simulink model "ferranti3phaseupfc41"  (R2016a)
settings: Solver=VariableStepAuto  StartTime=0.0  StopTime=10.0  RelTol=1e-3
undefined symbols (not defined in the file): D1, Delta
libraries: powerlib x20, powerlib_meascontrol x5, sps_avr x2, factslib x1
settings Model: Creator=prajay  LastModifiedBy=prajay

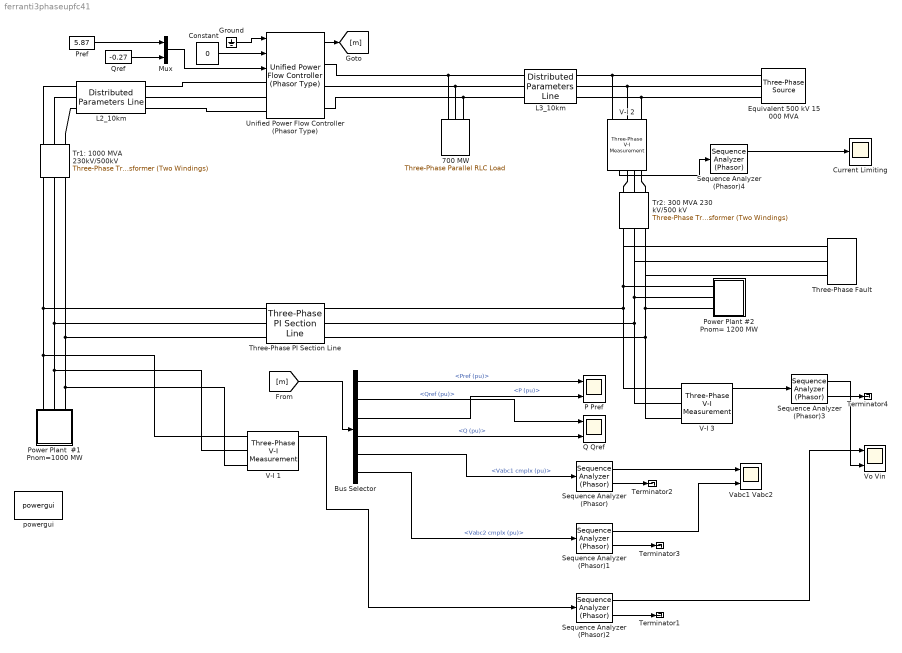
== system ferranti3phaseupfc41 ==
  700 MW : powerlib/Elements/Three-Phase Parallel RLC Load  LConnTagsString=A|B|C  Configuration=Y (grounded)  NominalVoltage=500e3  Vabc=[1e3 1e3 1e3]  Vabcp=[1e3 1e3 1e3]  NominalFrequency=60  UnbalancedPower=off  ActivePower=700e+006  InductivePower=0  CapacitivePower=0  Pabc=[10e3 9e3 11e3]  QLabc=[100 90 110]  QCabc=[100 90 110]  Pabcp=[10e3 9e3 11e3]  QLabcp=[100 90 110]  QCabcp=[100 90 110]  Measurements=None  LoadType=constant Z
  Bus Selector : BusSelector  OutputSignals=Control (Series).Pref (pu),Control (Series).Qref (pu),Control (Series).P (pu),Control (Series).Q (pu),Power.Vabc1 cmplx (pu),Power.Vabc2 cmplx (pu)
  Constant : Constant  Value=0
  Current Limiting : Scope
  Equivalent 500 kV 15 000 MVA : powerlib/Electrical Sources/Three-Phase Source  InternalConnection=Yg  VoltagePhases=off  Voltage=(500000)*1  PhaseAngle=3.2028e-005  Voltage_phases=[25e3 25e3 25e3]/sqrt(3)  PhaseAngles_phases=[0 -120 +120]  Frequency=60  NonIdealSource=on  SpecifyImpedance=on  Resistance=0.8929  Inductance=16.58e-3  ShortCircuitLevel=15000e6  BaseVoltage=500e3  XRratio=10  BusType=swing  Pref=0  Qref=0  Prefabc=0  Qrefabc=0  Qmin=-Inf  Qmax=Inf
  Ground : Ground
  L2_10km : powerlib/Elements/Distributed Parameters Line  Phases=3  Frequency=60  Resistance=[0.01273*2 0.3864]  Inductance="[0.9337e-3  4.1264e-3]"  Capacitance=[12.74e-9 7.751e-9]  Length=10  x1=[3.76470393664515e-08 500737.865699465 500737.698733622;376.991118430775 376.991118430775 376.991118430775;-1.76616198142372 0.572801869127968 -0.997994660183336]  x2=[3.31706486217144e-08 500303.506190995 500303.363079344;376.991118430775 376.991118430775 376.991118430775;-2.24825401600232 0.564569126636545 -1.00622737253496]  x3=[1.03911611711346e-09 676.330782319688 676.334945484693;376.991118430775 376.991118430775 376.991118430775;1.10566566451741 0.619123018648377 -0.951683326428739]  x4=[1.12477345287176e-09 3020.16196617448 3020.15620594757;376.991118430775 376.991118430775 376.991118430775;-2.03075400822802 0.549440453871556 -1.0213539651237]  x5=5.65541566995743e-05  V1=[3.169e-08 5.017e+05 5.017e+05;377 377 377;-0.2885 0.6054 -0.9654]  V2=[5.891e-08 5.011e+05 5.011e+05;377 377 377;2.202 0.568 -1.003]  I1=[1.07e-09 790.2 790.2;377 377 377;1.059 0.5023 -1.068]  I2=[1.028e-09 2904 2904;377 377 377;-2.11 0.5682 -1.003]  nHarmo=1  Measurements=Phase-to-ground voltages
      settings: AttributesFormatString=\n
  L3_10km : powerlib/Elements/Distributed Parameters Line  Phases=3  Frequency=60  Resistance=[0.01273*2 0.3864]  Inductance="[0.9337e-3  4.1264e-3]"  Capacitance=[12.74e-9 7.751e-9]  Length=10  x1=[3.32362335184301e-08 500303.388829253 500303.245718116;376.991118430775 376.991118430775 376.991118430775;-2.24805262409125 0.564569135773158 -1.00622736339962]  x2=[3.74559266249712e-08 500158.715856024 500158.596416031;376.991118430775 376.991118430775 376.991118430775;-2.6669204011152 0.566197665169602 -1.0045988035158]  x3=[9.25310885665503e-10 2074.37871582524 2074.38278202316;376.991118430775 376.991118430775 376.991118430775;1.21991146236643 0.586596456295587 -0.984203157060539]  x4=[9.8818528826696e-10 1620.48120507726 1620.47576843211;376.991118430775 376.991118430775 376.991118430775;-1.97224320713439 0.523398649863408 -1.04739401571321]  x5=5.65541566995743e-05  V1=[5.882e-08 5.011e+05 5.011e+05;377 377 377;2.203 0.568 -1.003]  V2=[1.45e-07 4.993e+05 4.993e+05;377 377 377;2.363 0.5448 -1.026]  I1=[1.123e-09 1185 1185;377 377 377;1.202 0.5674 -1.003]  I2=[1.02e-09 2501 2501;377 377 377;-2.175 0.5033 -1.068]  nHarmo=1  Measurements=None
      settings: AttributesFormatString=\n
  Mux : Mux  Inputs=2
  P Pref : Scope  NumInputPorts=2
  Power Plant  #1 Pnom=1000 MW : Subsystem
  Power Plant #2 Pnom= 1200 MW : Subsystem
  Pref : Constant  Value=5.87
  Q Qref : Scope  NumInputPorts=2
  Qref : Constant  Value=-0.27
  Sequence Analyzer (Phasor){,1..4} (5 alike) : powerlib_meascontrol/Measurements/Sequence Analyzer (Phasor)  seq=Positive
  Terminator{1..4} (4 alike) : Terminator
  Three-Phase PI Section Line : powerlib/Elements/Three-Phase PI Section Line  LConnTagsString=a|b|c  RConnTagsString=A|B|C  Frequency=60  Resistances=[ 0.01273 0.3864]  Inductances="[ 0.9337e-3  4.1264e-3]"  Capacitances=[12.74e-9 7.751e-9]  Length=800
  Three-Phase Fault : powerlib/Elements/Three-Phase Fault  InitialStates=0  FaultA=on  FaultB=on  FaultC=on  GroundFault=on  SwitchTimes="[1/60  5/60]"  External=off  SwitchStatus=NaN  FaultResistance=0.001  GroundResistance=0.01  SnubberResistance=1e6  SnubberCapacitance=inf  Measurements=None
  Tr1: 1000 MVA 230kV/500kV : powerlib/Elements/Three-Phase Transformer (Two Windings)  Winding1Connection=Yg  Winding2Connection=Yg  CoreType=Three single-phase transformers  SetSaturation=off  Hysteresis=off  DataFile='basic_model'  SetInitialFlux=off  Measurements=None  UNITS=pu  NominalPower=[ 1000e6 60 ]  Winding1="[ 230e3 0.002  0.0]"  Winding2=[ 500e3 0.002 0.12]  Rm=500  Lm=500  L0=0.5  Saturation="[ 0,0  ;  0.005,1.2  ;  1.0,1.4 ]"  InitialFluxes=[ 0.8 , -0.8 , 0.7 ]  MoreParameters=off  BreakLoop=off  DataType=off  TransfoNumber=0
  Tr2: 300 MVA 230 kV/500 kV : powerlib/Elements/Three-Phase Transformer (Two Windings)  Winding1Connection=Yg  Winding2Connection=Yg  CoreType=Three single-phase transformers  SetSaturation=off  Hysteresis=off  DataFile='basic_model'  SetInitialFlux=off  Measurements=Winding voltages  UNITS=pu  NominalPower=[ 300e6 60 ]  Winding1="[ 230e3 0.002  0.0]"  Winding2=[ 500e3 0.002 0.15]  Rm=500  Lm=500  L0=0.5  Saturation="[ 0,0  ;  0.005,1.2  ;  1.0,1.4 ]"  InitialFluxes=[ 0.8 , -0.8 , 0.7 ]  MoreParameters=off  BreakLoop=off  DataType=off  TransfoNumber=0
  Unified Power Flow Controller (Phasor Type) : factslib/Power-Electronics Based FACTS/Unified Power Flow Controller (Phasor Type)  SystemNominal=[ 500e3, 60 ]  Pnom_SH=100e6  RL_SH=[ 0.22/30, 0.22 ]  Iinit_SH=[0, 0 ]  SeriesNominal=[ 100e6, 0.1]  RL_SE=[ 0.16/30, 0.16 ]  Iinit_SE=[ 0 0]  VnomDC=40000  C_DC=1000e-6  OpMode_SH=Voltage regulation  Vref_SH=1.00  ExternalVref=off  MaxRateChangeVref_SH=0.1  Droop_SH=0.03  Par_VacReg=[5, 1000]  Qref_SH=0  MaxRateChangeQref_SH=2  Par_VdcReg=[0.1e-3, 20e-3]  Par_IReg_SH=[0.5, 25]/3  ExternalByPass=External control  OpMode_SE=Power flow control  PQref_SE=[5.87 -0.27]  ExternalPQref=on  Rate_PQref=1  Par_PReg_SE=[0.025, 1.5]  Vdqref_SE=[0.05, 0.05]  ExternalVdqref=off  Rate_Vdqref=0.2
  V-I 1 : powerlib/Measurements/Three-Phase V-I Measurement  VoltageMeasurement=phase-to-ground  SetLabelV=off  LabelV=Vabco  Vpu=on  VpuLL=off  CurrentMeasurement=yes  SetLabelI=off  LabelI=Iabco  Ipu=on  Pbase=100e6  Vbase=500e3  OutputType=Complex  PhasorSimulation=on  PSBequivalent=0
  V-I 2 : powerlib/Measurements/Three-Phase V-I Measurement  VoltageMeasurement=phase-to-ground  SetLabelV=off  LabelV=Vabco  Vpu=on  VpuLL=off  CurrentMeasurement=yes  SetLabelI=off  LabelI=Iabco  Ipu=on  Pbase=100e6  Vbase=500e3  OutputType=Complex  PhasorSimulation=on  PSBequivalent=0
  V-I 3 : powerlib/Measurements/Three-Phase V-I Measurement  VoltageMeasurement=phase-to-ground  SetLabelV=off  LabelV=Vabco  Vpu=on  VpuLL=off  CurrentMeasurement=yes  SetLabelI=off  LabelI=Iabco  Ipu=on  Pbase=100e6  Vbase=500e3  OutputType=Complex  PhasorSimulation=on  PSBequivalent=0
  Vabc1 Vabc2 : Scope  NumInputPorts=2
  Vo Vin : Scope  NumInputPorts=2
  powergui : powerlib/powergui  Priority=1  SimulationMode=Phasor  SolverType=Tustin/Backward Euler (TBE)  SampleTime=50e-6  frequency=60  SPID=off  DisableSnubberDevices=off  DisableRonSwitches=off  DisableVfSwitches=off  SwTol=0  DisplayEquations=off  Interpol=off  ExternalGateDelay=off  methode=off  Ts=10  FunctionMessages=off  echomessages=off  HookPort=off  EnableUseOfTLC=off  x0status=blocks  frequencyindice=60  Pbase=10e3  ErrMax=1e-4  Iterations=50  UnitsV=kV  UnitsW=MW  buscounter=0  RestoreLinks=warning  ResistiveCurrentMeasurement=off  Frange=[0:2:500]  Ylog=off  Xlog=on  ShowGrid=off  save=off  variable=ZData  structure=0  ZoomFFT=off  StartTime=0.0  cycles=1  DisplayStyle=1  fundamental=60  FreqAxis=off  MaxFrequency=1000  frequencyindicesteady=1  RmsSteady=2  display=off
  wires:
  Ground/1 -> Unified Power Flow Controller (Phasor Type)/1
  Mux/1 -> Unified Power Flow Controller (Phasor Type)/3
  Pref/1 -> Mux/1
  Qref/1 -> Mux/2
  Unified Power Flow Controller (Phasor Type)/1 -> [m]
  [m] -> Bus Selector/1
  Bus Selector/1 -> P Pref/1  "<Pref (pu)>"
  Bus Selector/2 -> Q Qref/1  "<Qref (pu)>"
  Bus Selector/3 -> P Pref/2  "<P (pu)>"
  Bus Selector/4 -> Q Qref/2  "<Q (pu)>"
  Bus Selector/5 -> Sequence Analyzer (Phasor)/1  "<Vabc1 cmplx (pu)>"
  Bus Selector/6 -> Sequence Analyzer (Phasor)1/1  "<Vabc2 cmplx (pu)>"
  V-I 1/1 -> Sequence Analyzer (Phasor)2/1
  Sequence Analyzer (Phasor)1/2 -> Terminator3/1
  Sequence Analyzer (Phasor)2/2 -> Terminator1/1
  Sequence Analyzer (Phasor)/2 -> Terminator2/1
  Sequence Analyzer (Phasor)3/2 -> Terminator4/1
  Sequence Analyzer (Phasor)2/1 -> Vo Vin/1
  Sequence Analyzer (Phasor)3/1 -> Vo Vin/2
  V-I 3/1 -> Sequence Analyzer (Phasor)3/1
  Sequence Analyzer (Phasor)/1 -> Vabc1 Vabc2/1
  Sequence Analyzer (Phasor)1/1 -> Vabc1 Vabc2/2
  V-I 2/2 -> Sequence Analyzer (Phasor)4/1
  Sequence Analyzer (Phasor)4/1 -> Current Limiting/1
  Constant/1 -> Unified Power Flow Controller (Phasor Type)/2
  connections:
  V-I 3/LConn3 -- Tr2: 300 MVA 230 kV/500 kV/LConn3 -- Three-Phase Fault/LConn3 -- Power Plant #2 Pnom= 1200 MW/RConn3 -- Three-Phase PI Section Line/RConn3
  L3_10km/LConn1 -- Unified Power Flow Controller (Phasor Type)/RConn1 -- 700 MW/LConn1
  L2_10km/RConn1 -- Unified Power Flow Controller (Phasor Type)/LConn1
  L2_10km/RConn2 -- Unified Power Flow Controller (Phasor Type)/LConn2
  L3_10km/LConn2 -- 700 MW/LConn2 -- Unified Power Flow Controller (Phasor Type)/RConn2
  Three-Phase PI Section Line/LConn1 -- Tr1: 1000 MVA 230kV/500kV/LConn1 -- V-I 1/LConn1 -- Power Plant  #1 Pnom=1000 MW/RConn1
  Three-Phase PI Section Line/LConn3 -- Tr1: 1000 MVA 230kV/500kV/LConn3 -- V-I 1/LConn3 -- Power Plant  #1 Pnom=1000 MW/RConn3
  Unified Power Flow Controller (Phasor Type)/LConn3 -- L2_10km/RConn3
  700 MW/LConn3 -- L3_10km/LConn3 -- Unified Power Flow Controller (Phasor Type)/RConn3
  Three-Phase PI Section Line/LConn2 -- Tr1: 1000 MVA 230kV/500kV/LConn2 -- V-I 1/LConn2 -- Power Plant  #1 Pnom=1000 MW/RConn2
  L3_10km/RConn1 -- Equivalent 500 kV 15 000 MVA/RConn1 -- V-I 2/LConn1
  L3_10km/RConn2 -- Equivalent 500 kV 15 000 MVA/RConn2 -- V-I 2/LConn2
  L3_10km/RConn3 -- Equivalent 500 kV 15 000 MVA/RConn3 -- V-I 2/LConn3
  Tr1: 1000 MVA 230kV/500kV/RConn1 -- L2_10km/LConn1
  Tr1: 1000 MVA 230kV/500kV/RConn2 -- L2_10km/LConn2
  Tr1: 1000 MVA 230kV/500kV/RConn3 -- L2_10km/LConn3
  V-I 3/LConn1 -- Tr2: 300 MVA 230 kV/500 kV/LConn1 -- Three-Phase Fault/LConn1 -- Power Plant #2 Pnom= 1200 MW/RConn1 -- Three-Phase PI Section Line/RConn1
  V-I 3/LConn2 -- Tr2: 300 MVA 230 kV/500 kV/LConn2 -- Three-Phase Fault/LConn2 -- Power Plant #2 Pnom= 1200 MW/RConn2 -- Three-Phase PI Section Line/RConn2
  V-I 2/RConn1 -- Tr2: 300 MVA 230 kV/500 kV/RConn1
  V-I 2/RConn2 -- Tr2: 300 MVA 230 kV/500 kV/RConn2
  V-I 2/RConn3 -- Tr2: 300 MVA 230 kV/500 kV/RConn3

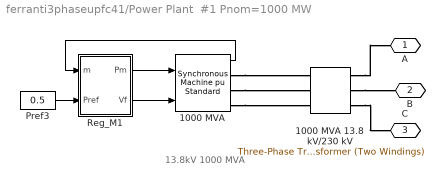
== system ferranti3phaseupfc41/Power Plant  #1 Pnom=1000 MW ==
  note: 13.8kV 1000 MVA
  1000 MVA : powerlib/Machines/Synchronous Machine pu Standard  PresetModel=No  MechanicalLoad=Mechanical power Pm  ShowDetailedParameters=on  RotorType=Salient-pole  Units=per unit standard parameters  MeasurementBus=off  NominalParameters="[1000E6  13800   60 ]"  Reactances1=[ 31 32 33 34 35 36 37 ]  Reactances2=[ 1.305, 0.296, 0.252, 0.474, 0.243, 0.18 ]  dAxisTimeConstants=Short-circuit  qAxisTimeConstants=Open-circuit  TimeConstants1=[]  TimeConstants2=[]  TimeConstants3=[]  TimeConstants4=[]  TimeConstants5=[ 1.01, 0.053, 0.1 ]  TimeConstants6=[]  TimeConstants7=[]  TimeConstants8=[]  StatorResistance=2.8544e-3  Mechanical="[ 3.7 0  32]"  PolePairs=32  InitialConditions=[0 -90.4528 0.500842 0.500842 0.500842 -16.9126 -136.913 103.087 1.1604]  SetSaturation=off  Saturation=[0.6404,0.7127,0.8441,0.9214,0.9956,1.082,1.19,1.316,1.457;0.7,0.7698,0.8872,0.9466,0.9969,1.046,1.1,1.151,1.201]  LoadFlowParameters=[1 500000000 0 0 0]  TsPowergui=0  TsBlock=-1  IterativeModel=Trapezoidal non iterative  IterativeDiscreteModel=Trapezoidal non iterative  BusType=PV  Pref=5e+008  Qref=0  Qmin=-Inf  Qmax=Inf  PLF=0  QLF=0
      settings: AttributesFormatString=\n\n
  1000 MVA 13.8 kV/230 kV : powerlib/Elements/Three-Phase Transformer (Two Windings)  Winding1Connection=Delta (D1)  Winding2Connection=Yg  CoreType=Three single-phase transformers  SetSaturation=off  Hysteresis=off  DataFile='basic_model'  SetInitialFlux=off  Measurements=None  UNITS=pu  NominalPower=[ 1000e6 60 ]  Winding1="[ 13.8e3 0.002  0.0]"  Winding2=[ 230e3 0.002 0.12]  Rm=500  Lm=500  L0=0.5  Saturation="[ 0,0  ;  0.005,1.2  ;  1.0,1.4 ]"  InitialFluxes=[ 0.8 , -0.8 , 0.7 ]  MoreParameters=off  BreakLoop=off  DataType=off  TransfoNumber=0
  Pref3 : Constant  Value=0.5
  Reg_M1 : Subsystem
  A : PMIOPort  Port=1  Side=Right
  B : PMIOPort  Port=2  Side=Right
  C : PMIOPort  Port=3  Side=Right
  wires:
  Reg_M1/1(Pm) -> 1000 MVA/1
  Reg_M1/2(Vf) -> 1000 MVA/2
  Pref3/1 -> Reg_M1/2(Pref)
  1000 MVA/1 -> Reg_M1/1(m)
  connections:
  1000 MVA/RConn1 -- 1000 MVA 13.8 kV/230 kV/LConn1
  1000 MVA/RConn2 -- 1000 MVA 13.8 kV/230 kV/LConn2
  1000 MVA/RConn3 -- 1000 MVA 13.8 kV/230 kV/LConn3
  1000 MVA 13.8 kV/230 kV/RConn1 -- A/RConn1
  1000 MVA 13.8 kV/230 kV/RConn2 -- B/RConn1
  1000 MVA 13.8 kV/230 kV/RConn3 -- C/RConn1

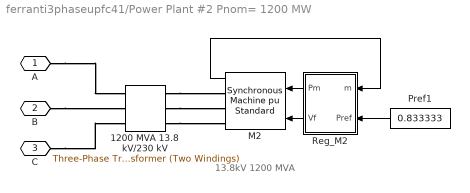
== system ferranti3phaseupfc41/Power Plant #2 Pnom= 1200 MW ==
  note: 13.8kV 1200 MVA
  1200 MVA 13.8 kV/230 kV : powerlib/Elements/Three-Phase Transformer (Two Windings)  Winding1Connection=Delta (D1)  Winding2Connection=Yg  CoreType=Three single-phase transformers  SetSaturation=off  Hysteresis=off  DataFile='basic_model'  SetInitialFlux=off  Measurements=None  UNITS=pu  NominalPower=[ 1200e6 60 ]  Winding1="[ 13.8e3 0.002  0.0]"  Winding2=[ 230e3 0.002 0.12]  Rm=500  Lm=500  L0=0.5  Saturation="[ 0,0  ;  0.005,1.2  ;  1.0,1.4 ]"  InitialFluxes=[ 0.8 , -0.8 , 0.7 ]  MoreParameters=off  BreakLoop=off  DataType=off  TransfoNumber=0
  M2 : powerlib/Machines/Synchronous Machine pu Standard  PresetModel=No  MechanicalLoad=Mechanical power Pm  ShowDetailedParameters=on  RotorType=Salient-pole  Units=per unit standard parameters  MeasurementBus=off  NominalParameters="[1200E6  13800   60 ]"  Reactances1=[ 31 32 33 34 35 36 37 ]  Reactances2=[ 1.305, 0.296, 0.252, 0.474, 0.243, 0.18 ]  dAxisTimeConstants=Short-circuit  qAxisTimeConstants=Open-circuit  TimeConstants1=[]  TimeConstants2=[]  TimeConstants3=[]  TimeConstants4=[]  TimeConstants5=[ 1.01, 0.053, 0.1 ]  TimeConstants6=[]  TimeConstants7=[]  TimeConstants8=[]  StatorResistance=2.8544e-3  Mechanical="[ 3.7 0  32]"  PolePairs=32  InitialConditions=[0 -78.7337 0.836975 0.836975 0.836975 -14.879 -134.879 105.121 1.41828]  SetSaturation=off  Saturation=[0.6404,0.7127,0.8441,0.9214,0.9956,1.082,1.19,1.316,1.457;0.7,0.7698,0.8872,0.9466,0.9969,1.046,1.1,1.151,1.201]  LoadFlowParameters=[1 1000000000 0 0 0]  TsPowergui=0  TsBlock=-1  IterativeModel=Trapezoidal non iterative  IterativeDiscreteModel=Trapezoidal non iterative  BusType=PV  Pref=1e+009  Qref=0  Qmin=-Inf  Qmax=Inf  PLF=0  QLF=0
      settings: AttributesFormatString=\n\n
  Pref1 : Constant  Value=0.833333
  Reg_M2 : Subsystem
  A : PMIOPort  Port=1  Side=Right
  B : PMIOPort  Port=2  Side=Right
  C : PMIOPort  Port=3  Side=Right
  wires:
  Reg_M2/1(Pm) -> M2/1
  Reg_M2/2(Vf) -> M2/2
  Pref1/1 -> Reg_M2/2(Pref)
  M2/1 -> Reg_M2/1(m)
  connections:
  1200 MVA 13.8 kV/230 kV/LConn1 -- M2/RConn1
  1200 MVA 13.8 kV/230 kV/LConn2 -- M2/RConn2
  1200 MVA 13.8 kV/230 kV/LConn3 -- M2/RConn3
  A/RConn1 -- 1200 MVA 13.8 kV/230 kV/RConn1
  B/RConn1 -- 1200 MVA 13.8 kV/230 kV/RConn2
  C/RConn1 -- 1200 MVA 13.8 kV/230 kV/RConn3

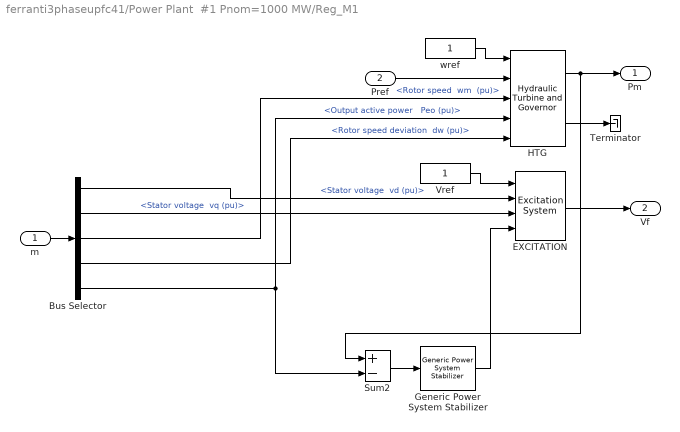
== system ferranti3phaseupfc41/Power Plant  #1 Pnom=1000 MW/Reg_M1 ==
  m : Inport
  Pref : Inport  Port=2
  Bus Selector : BusSelector  OutputSignals="dq0 components.Stator voltage  vd (pu),dq0 components.Stator voltage  vq (pu),Mechanical.Rotor speed  wm  (pu),Mechanical.Rotor speed deviation  dw (pu),Output active power   Peo (pu)"
  EXCITATION : sps_avr/Excitation System  tr=20e-3  reg=[ 200, 0.001 ]  exc=[ 1, 0 ]  tgr=[ 0, 0 ]  damp=[ 0.001, 0.1 ]  sat=[ 0, 0 ]  lim="[ 0,  7, 0 ]"  v0=[1,1.1604]
  Generic Power System Stabilizer : powerlib/Machines/Generic Power System Stabilizer  Tsensor=15e-3  K=2.5  Twashout=1  Tleadlag1="[0.06  1]"  Tleadlag2="[0  0]"  VSlimits=[-0.15 0.15]  Vinit=0  Plot_On=off  MagdB_On=on  FreqRange=logspace(-2,2,500)
  HTG : powerlib/Machines/Hydraulic Turbine and Governor  sm="[ 10/3  0.07 ]"  gate="[  0.01  0.97518  -0.1  0.1 ]"  reg="[  0.05  1.163  0.105  0  0.01  ]"  hyd="[  0  2.67  ]"  dref=0  po=0.500716
  Sum2 : Sum  Inputs=+-  SaturateOnIntegerOverflow=on  InputSameDT=on  OutDataTypeStr=Inherit: Same as first input
  Terminator : Terminator
  Vref : Constant
  wref : Constant
  Pm : Outport  InitialOutput=0
  Vf : Outport  Port=2  InitialOutput=0
  wires:
  HTG/2 -> Terminator/1
  Vref/1 -> EXCITATION/1
  m/1 -> Bus Selector/1
  Bus Selector/4 -> HTG/5  "<Rotor speed deviation  dw (pu)>"
  Bus Selector/5 -> HTG/4, Sum2/2  "<Output active power   Peo (pu)>"
  Bus Selector/3 -> HTG/3  "<Rotor speed  wm  (pu)>"
  Pref/1 -> HTG/2
  wref/1 -> HTG/1
  HTG/1 -> Pm/1, Sum2/1
  Bus Selector/2 -> EXCITATION/3  "<Stator voltage  vq (pu)>"
  EXCITATION/1 -> Vf/1
  Bus Selector/1 -> EXCITATION/2  "<Stator voltage  vd (pu)>"
  Generic Power System Stabilizer/1 -> EXCITATION/4
  Sum2/1 -> Generic Power System Stabilizer/1

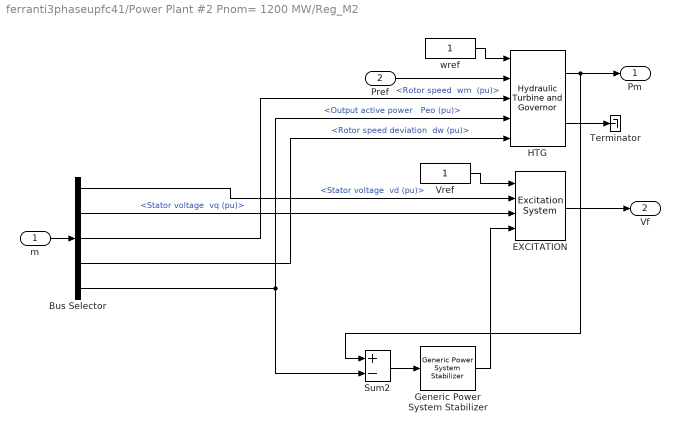
== system ferranti3phaseupfc41/Power Plant #2 Pnom= 1200 MW/Reg_M2 ==
  m : Inport
  Pref : Inport  Port=2
  Bus Selector : BusSelector  OutputSignals="dq0 components.Stator voltage  vd (pu),dq0 components.Stator voltage  vq (pu),Mechanical.Rotor speed  wm  (pu),Mechanical.Rotor speed deviation  dw (pu),Output active power   Peo (pu)"
  EXCITATION : sps_avr/Excitation System  tr=20e-3  reg=[ 200, 0.001 ]  exc=[ 1, 0 ]  tgr=[ 0, 0 ]  damp=[ 0.001, 0.1 ]  sat=[ 0, 0 ]  lim="[ 0,  7, 0 ]"  v0=[1,1.41828]
  Generic Power System Stabilizer : powerlib/Machines/Generic Power System Stabilizer  Tsensor=15e-3  K=2.5  Twashout=1  Tleadlag1="[0.06  1]"  Tleadlag2="[0  0]"  VSlimits=[-0.15 0.15]  Vinit=0  Plot_On=off  MagdB_On=on  FreqRange=logspace(-2,2,500)
  HTG : powerlib/Machines/Hydraulic Turbine and Governor  sm="[ 10/3  0.07 ]"  gate="[  0.01  0.97518  -0.1  0.1 ]"  reg="[  0.05  1.163  0.105  0  0.01  ]"  hyd="[  0  2.67  ]"  dref=0  po=0.835333
  Sum2 : Sum  Inputs=+-  SaturateOnIntegerOverflow=on  InputSameDT=on  OutDataTypeStr=Inherit: Same as first input
  Terminator : Terminator
  Vref : Constant
  wref : Constant
  Pm : Outport  InitialOutput=0
  Vf : Outport  Port=2  InitialOutput=0
  wires:
  HTG/2 -> Terminator/1
  Vref/1 -> EXCITATION/1
  m/1 -> Bus Selector/1
  Bus Selector/4 -> HTG/5  "<Rotor speed deviation  dw (pu)>"
  Bus Selector/5 -> HTG/4, Sum2/2  "<Output active power   Peo (pu)>"
  Bus Selector/3 -> HTG/3  "<Rotor speed  wm  (pu)>"
  Pref/1 -> HTG/2
  wref/1 -> HTG/1
  HTG/1 -> Pm/1, Sum2/1
  Bus Selector/2 -> EXCITATION/3  "<Stator voltage  vq (pu)>"
  EXCITATION/1 -> Vf/1
  Bus Selector/1 -> EXCITATION/2  "<Stator voltage  vd (pu)>"
  Generic Power System Stabilizer/1 -> EXCITATION/4
  Sum2/1 -> Generic Power System Stabilizer/1
